simulink model "traj_model"  (R2022b)
settings: Solver=VariableStepAuto  StartTime=0.0  StopTime=600  RelTol=1e-3
values from neighbouring files (symbols this model uses):
  L = 235    [trajectory_script.m]
settings Model: Creator=hamra  LastModifiedBy=hamra

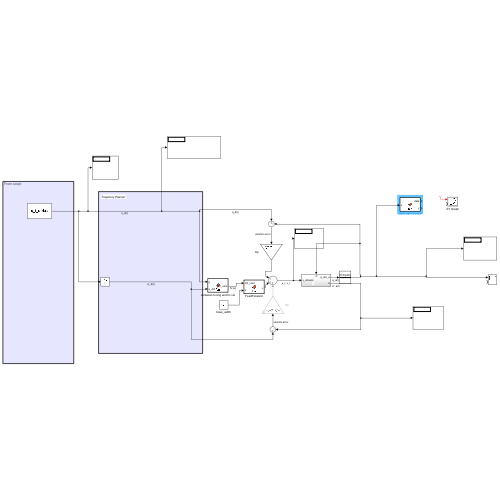
[thumbnail: Simulink's stored preview of the top-level diagram]
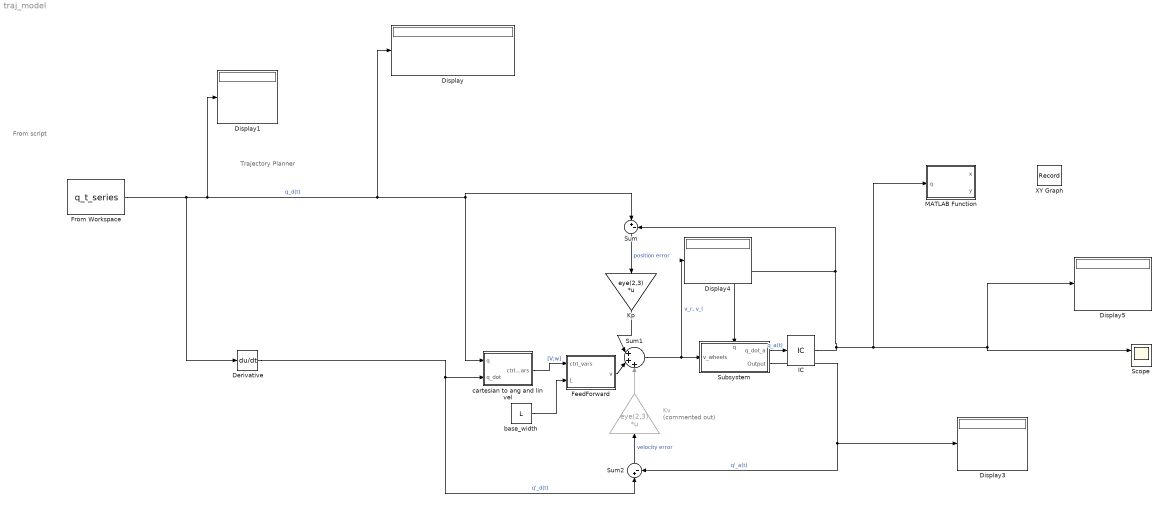
== system traj_model ==
  note: From script
  note: Trajectory Planner
  Derivative : Derivative
  Display{,1,3..5} (5 alike) : Display
  FeedForward : MATLAB Function  TreatAsAtomicUnit=on
  From Workspace : FromWorkspace  VariableName=q_t_series
  IC : InitialCondition  Value=[0;0;pi/4]
  Kp : Gain  Gain=eye(2,3)  Multiplication=Matrix(K*u)
  Kv : Gain  Commented=on  Gain=eye(2,3)  Multiplication=Matrix(K*u)
  MATLAB Function : MATLAB Function  TreatAsAtomicUnit=on
  Scope : Scope  NumInputPorts=2
  Subsystem : Subsystem
      settings: PortSchema="{\"entries\":[{\"content\":{\"sides\":[{\"content\":{\"connectorIds\":[\"In1\"]},\"type\":\"ConnectorPlacement.EquallySpacedRectSide\",\"uuid\":\"55772681-8002-4081-a158-24497c876b6c\"},{\"content\":{\"connectorIds\":[\"Out1\",\"Out2\"],\"side\":\"RIGHT\"},\"type\":\"ConnectorPlacement.EquallySpacedRectSide\",\"uuid\":\"cbc9689a-22e5-459f-948c-5dae70d8c4ac\"},{\"content\":{\"connectorIds\":[\"In2\"],\"side\":\"TOP\"},\"type\":\"ConnectorPlacement.EquallySpacedRectSide\",\"uuid\":\"37c3a931-4b64-4e59-91ae-4b6fdc9d9254\"}]},\"type\":\"ConnectorPlacement.EquallySpacedConnector\",\"uuid\":\"5e43323b-0ad5-4079-b895-b0c0c428e1c7\"}],\"packageUris\":[\"http://schema.mathworks.com/mf0/Connector/R2020b\"],\"version\":\"1.0\"}"
  Sum : Sum  Inputs=|+-
  Sum1 : Sum  Inputs=|+++
  Sum2 : Sum  Inputs=|+-
  XY Graph : Record  FileSettingsInternal="{\"entries\":[{\"content\":{\"excelSettings\":{\"content\":{},\"type\":\"Streamout.ExcelSettings\"}},\"type\":\"Streamout.FileSettingStorage\",\"uuid\":\"58ab379a-1777-4653-92fb-12abd4dd8c21\"}],\"packageUris\":[\"http://schema.mathworks.com/mf0/streamout_blocks/R2020a\"],\"version\":\"1.0\"}"  Layout=[1 1]  SignalsInternal="{\"entries\":[{\"content\":{\"signals\":[{\"content\":{\"blockPath\":[\"traj_model/XY Graph\"],\"channel\":[],\"dimensions\":[1],\"domain\":\"traj_model/XY Graph\",\"lineColor\":\"#a2142f\",\"plots\":[1],\"port\":1,\"sid\":[],\"signalID\":16,\"signalName\":\"XY Graph:1\"},\"type\":\"RecordBlkView.Signal\",\"uuid\":\"ab7b26d7-c70f-4fb9-803b-bdde5512abf3\"},{\"content\":{\"blockPath\":[\"traj_model/XY Graph\"],\"channel\":[],\"dimensions\":[1],\"domain\":\"traj_model/XY Graph\",\"lineColor\":\"#139fff\",\"plots\":[1],\"port\":2,\"sid\":[],\"signalID\":19,\"signalName\":\"XY Graph:2\"},\"type\":\"RecordBlkView.Signal\",\"uuid\":\"25b8a358-cc35-4a2c-8b11-659c8d0ff94a\"}]},\"type\":\"RecordBlkView.InputSignals\",\"uuid\":\"38969fe3-63cc-42af-837d-76ca5558e862\"}],\"packageUris\":[\"http://schema.mathworks.com/mf0/streamout_blocks/R2020a\"],\"version\":\"1.0\"}"  VisualizationBindings="{\"xyplotplugin\":{\"info\":[{\"series\":[{\"bindingParametersList\":[{\"parameter\":\"X-Axis\",\"signalID\":16,\"signalName\":\"XY Graph:1\"},{\"parameter\":\"Y-Axis\",\"signalID\":19,\"signalName\":\"XY Graph:2\"}],\"seriesID\":25269}],\"subplotID\":1}]}}"  CompatibilityTag=XY
  base_width : Constant  Value=L
  cartesian to ang and lin vel : MATLAB Function  TreatAsAtomicUnit=on
  wires:
  Kp/1 -> Sum1/1
  Sum/1 -> Kp/1  "position error"
  Kv/1 -> Sum1/3
  Sum2/1 -> Kv/1  "velocity error"
  From Workspace/1 -> Display1/1, Display/1, Sum/1, cartesian to ang and lin vel/1(q), Derivative/1  "q_d(t)"
  Sum1/1 -> Display4/1, Subsystem/1(v_wheels)  "v_r, v_l"
  FeedForward/1(v) -> Sum1/2
  Subsystem/1(q_dot_a) -> IC/1  "q_a(t)"
  Derivative/1 -> Sum2/1, cartesian to ang and lin vel/2(q_dot)  "q'_d(t)"
  Subsystem/2(Output) -> Sum2/2, Display3/1  "q'_a(t)"
  cartesian to ang and lin vel/1(ctrl_vars) -> FeedForward/1(ctrl_vars)  "[V;w]"
  base_width/1 -> FeedForward/2(L)
  IC/1 -> MATLAB Function/1(q), Display5/1, Scope/1, Subsystem/2(q), Sum/2
  ? -> XY Graph/1

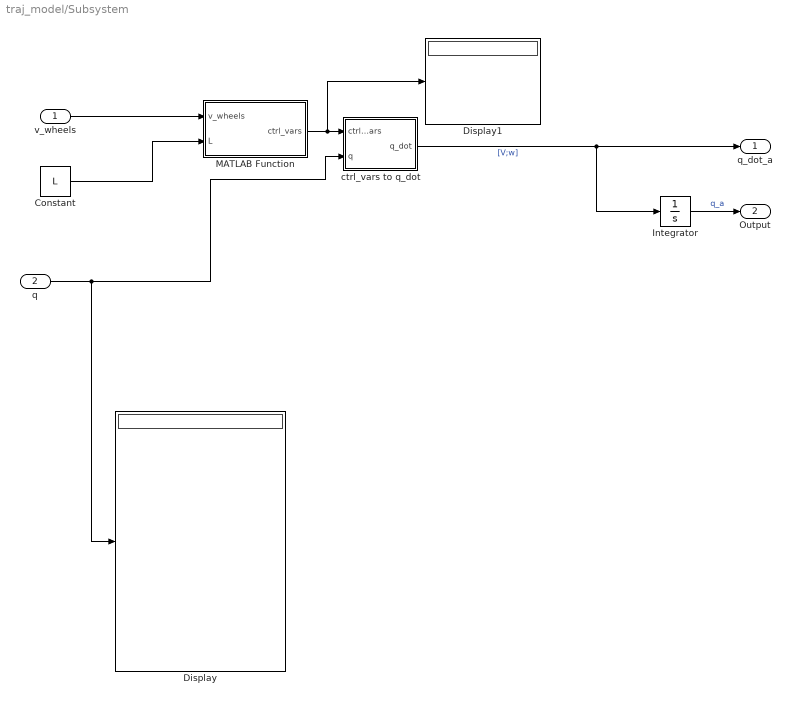
== system traj_model/Subsystem ==
  v_wheels : Inport
  q : Inport  Port=2
  Constant : Constant  Value=L
  Display : Display
  Display1 : Display
  Integrator : Integrator
  MATLAB Function : MATLAB Function  TreatAsAtomicUnit=on
  ctrl_vars to q_dot : MATLAB Function  TreatAsAtomicUnit=on
  q_dot_a : Outport
  Output : Outport  Port=2
  wires:
  Integrator/1 -> Output/1  "q_a"
  v_wheels/1 -> MATLAB Function/1(v_wheels)
  Constant/1 -> MATLAB Function/2(L)
  q/1 -> Display/1, ctrl_vars to q_dot/2(q)
  ctrl_vars to q_dot/1(q_dot) -> Integrator/1, q_dot_a/1  "[V;w]"
  MATLAB Function/1(ctrl_vars) -> Display1/1, ctrl_vars to q_dot/1(ctrl_vars)

== matlab function traj_model/cartesian to ang and lin vel ==
  data: q input; q_dot input; ctrl_vars output
function ctrl_vars = fcn(q,q_dot)
theta = q(3);
T = [cos(theta) 0; sin(theta) 0; 0 1];

ctrl_vars = pinv(T)*q_dot;

== matlab function traj_model/Subsystem/MATLAB Function ==
  data: v_wheels input; ctrl_vars output; L input
function ctrl_vars = fcn(v_wheels, L)

T = 1/2*[1 1 ; 1/L -1/L];

ctrl_vars = pinv(T)*v_wheels;

== matlab function traj_model/Subsystem/ctrl_vars to q_dot ==
  data: ctrl_vars input; q_dot output; q input
function q_dot = fcn(ctrl_vars,q)
theta = q(3);
T = [cos(theta) 0; sin(theta) 0; 0 1];

q_dot =  T*ctrl_vars;

== matlab function traj_model/MATLAB Function ==
  data: x output; q input; y output
function [x, y]= fcn(q)
x = q(1);
y = q(2);

== matlab function traj_model/FeedForward ==
  data: ctrl_vars input; v output; L input
function v = fcn(ctrl_vars,L)
%L = 235; %nominal base width [mm]


w = ctrl_vars(2); 
V = ctrl_vars(1);

v_1 = V + L/2*w; %right velocity [mm/s]
v_2 = V - L/2*w; %left velocity [mm/s]
v = [v_1;v_2]; %velocity vector
